simulink subsystem "Sub_Reference_parameters"  (R2020a)
settings: Solver=VariableStepAuto  StartTime=0.0  StopTime=10.0  RelTol=1e-3
settings Model: Creator=Lamarre  LastModifiedBy=Lamarre

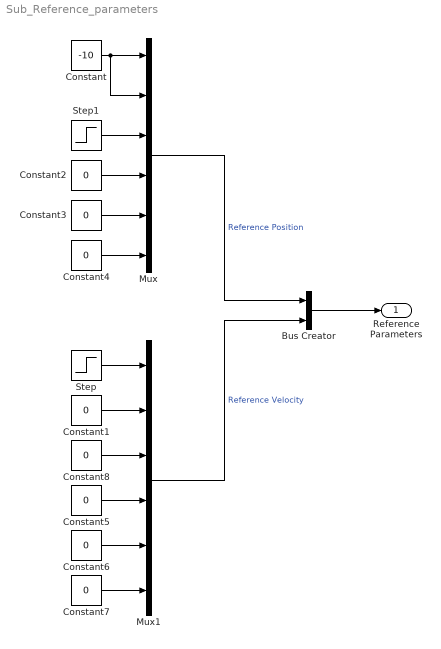
== system Sub_Reference_parameters ==
  Bus Creator : BusCreator  Inputs=2
  Constant : Constant  Value=-10
  Constant{1..8} (8 alike) : Constant  Value=0
  Mux : Mux  Inputs=6
  Mux1 : Mux  Inputs=6
  Step : Step  Time=30  Before=0.2  After=0  SampleTime=0
  Step1 : Step  Time=150  After=5  SampleTime=0
  Reference Parameters : Outport  VectorParamsAs1DForOutWhenUnconnected=off
  wires:
  Constant5/1 -> Mux1/4
  Constant7/1 -> Mux1/6
  Constant3/1 -> Mux/5
  Constant2/1 -> Mux/4
  Step/1 -> Mux1/1
  Mux1/1 -> Bus Creator/2  "Reference Velocity"
  Constant/1 -> Mux/2, Mux/1
  Bus Creator/1 -> Reference Parameters/1
  Mux/1 -> Bus Creator/1  "Reference Position"
  Constant6/1 -> Mux1/5
  Constant1/1 -> Mux1/2
  Step1/1 -> Mux/3
  Constant4/1 -> Mux/6
  Constant8/1 -> Mux1/3
